simulink model "NewModel_v2"  (R2020a)
settings: Solver=VariableStepAuto  StartTime=0.0  StopTime=1000  FixedStep=0.1  RelTol=1e-3
values from neighbouring files (symbols this model uses):
  Ctr = 1.6    [ACC_DATA.m]
  F_aero = 1/(2*m_Follower)*Ro_A_Cd    (= 0.00026)    [ACC_DATA.m]
  F_grav = g*sin(theta)    [ACC_DATA.m]
  F_res = g*Cr*cos(theta)    [ACC_DATA.m]
  Kb = 0.08    [ACC_DATA.m]
  Kc = 1    [ACC_DATA.m]
  m_Follower = 1500    [ACC_DATA.m]
  max_ac = 3    [ACC_DATA.m]
  min_ac = -3    [ACC_DATA.m]
  r = 0.326    [ACC_DATA.m]
  Rf = 3.28    [ACC_DATA.m]
  Rtr = 1    [ACC_DATA.m]
  Tmax = 528.7 + 0.152*Ne - 0.0000217*Ne^2    (= 789.5)    [ACC_DATA.m]
  Ts = 0.1    [ACC_DATA.m]
  v0_lead = 20    [ACC_DATA.m]
  verr_gain = 0.4    [ACC_DATA.m]
  vx_gain = 0.1    [ACC_DATA.m]
  x0_ego = 10    [ACC_DATA.m]
  x0_lead = 500    [ACC_DATA.m]
  xerr_gain = 0.8    [ACC_DATA.m]
undefined symbols (not defined in the file or in its folder): sigbuilder_block
libraries: simulink x5
settings Model: SimulationMode=accelerator  Creator=91968  LastModifiedBy=91968

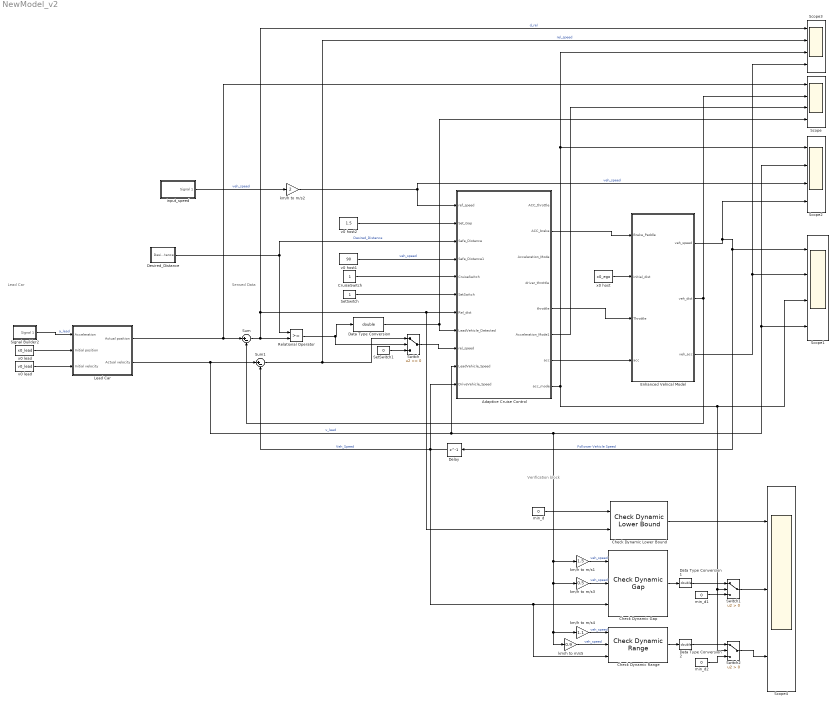
== system NewModel_v2 ==
  note: Verification block
  note: Lead Car
  note: Sensed Data
  Adaptive Cruise Control : Subsystem
  Check Dynamic Gap : simulink/Model Verification/Check  Dynamic Gap  Description=u < min || max < u  enabled=on  stopWhenAssertionFail=off  export=on  icon=graphic
      settings: SourceProductBaseCode=SL
  Check Dynamic Range : simulink/Model Verification/Check  Dynamic Range  Description=min < u < max  enabled=on  stopWhenAssertionFail=off  export=on  icon=graphic
      settings: SourceProductBaseCode=SL
  Check Dynamic Lower Bound : simulink/Model Verification/Check Dynamic  Lower Bound  Description=min < u  Enabled=on  stopWhenAssertionFail=off  export=on  icon=graphic
      settings: SourceProductBaseCode=SL
  CruiseSwitch : Constant
  Data Type Conversion : DataTypeConversion  OutDataTypeStr=double
  Data Type Conversion1 : DataTypeConversion  OutDataTypeStr=double
  Data Type Conversion2 : DataTypeConversion  OutDataTypeStr=double
  Delay : Delay  DelayLength=1  InitialCondition=0
  Desired_Distance : Subsystem  mask{Desired_Distance=10.0}
      mask DialogControl DescGroupVar Prompt: Set Desired Distance
      mask Display: image('C:\Users\Talha Rao\Pictures\070558928_iconm (2).jpeg');
  Enhanced Vehical Model : Subsystem
  Lead Car : Subsystem
  Relational Operator : RelationalOperator  OutDataTypeStr=boolean  RndMeth=Simplest
  Scope{,1..3} (4 alike) : Scope  NumInputPorts=4
  Scope4 : Scope  NumInputPorts=3
  SetSwitch : Constant
  SetSwitch1 : Constant  Value=0
  Signal Builder2 : Subsystem  Tag=STV Subsys  LoadFcn=sigbuilder_block('load');  StartFcn=sigbuilder_block('start');  StopFcn=sigbuilder_block('stop');  ClipboardFcn=sigbuilder_block('clipboard');  mask(Sigbuilder block){tuvar=[0:10]}
      mask help: Simulink:masks:SigbuilderBlock_MD
      mask init:
      | if ~strcmp(get_param(bdroot(gcbh),'SimulationStatus'),'stopped') tuvar = sigbuilder_block('maskInit'); end
      settings: CopyFcn=sigbuilder_block('copy');  DeleteFcn=sigbuilder_block('delete');  ModelCloseFcn=sigbuilder_block('modelClose');  PreSaveFcn=sigbuilder_block('preSave');  PauseFcn=sigbuilder_block('pause');  ContinueFcn=sigbuilder_block('continue');  NameChangeFcn=sigbuilder_block('namechange');  OpenFcn=sigbuilder_block('open',[-1359 225 891.75 468.75 ]);  CloseFcn=sigbuilder_block('close');
      mask Display: plot(0, 0, 100, 100,[2, 2, 32, 32, 2], [68, 8, 8, 68, 68],[32, 2], [38, 38], [32, 19, 2],[53, 60, 44], [32, 17, 17, 2],[16, 16, 31, 31]);txt = getActiveGroup(gcbh);text(2, 100, txt,'verticalAlignment', 'top');
  Sum : Sum  Inputs=|+-
  Sum1 : Sum  Inputs=|+-
  Switch : Switch  SaturateOnIntegerOverflow=on  InputSameDT=on
  Switch1 : Switch  Criteria=u2 > Threshold  SaturateOnIntegerOverflow=on  InputSameDT=on
  Switch2 : Switch  Criteria=u2 > Threshold  SaturateOnIntegerOverflow=on  InputSameDT=on
  input_speed : Subsystem  Tag=STV Subsys  LoadFcn=sigbuilder_block('load');  StartFcn=sigbuilder_block('start');  StopFcn=sigbuilder_block('stop');  ClipboardFcn=sigbuilder_block('clipboard');  mask(Sigbuilder block){tuvar=[0:10]}
      mask help: Simulink:masks:SigbuilderBlock_MD
      mask init:
      | if ~strcmp(get_param(bdroot(gcbh),'SimulationStatus'),'stopped') tuvar = sigbuilder_block('maskInit'); end
      settings: CopyFcn=sigbuilder_block('copy');  DeleteFcn=sigbuilder_block('delete');  ModelCloseFcn=sigbuilder_block('modelClose');  PreSaveFcn=sigbuilder_block('preSave');  PauseFcn=sigbuilder_block('pause');  ContinueFcn=sigbuilder_block('continue');  NameChangeFcn=sigbuilder_block('namechange');  OpenFcn=sigbuilder_block('open',[0 36 1440 716.25 ]);  CloseFcn=sigbuilder_block('close');
      mask Display: plot(0, 0, 100, 100,[2, 2, 32, 32, 2], [68, 8, 8, 68, 68],[32, 2], [38, 38], [32, 19, 2],[53, 60, 44], [32, 17, 17, 2],[16, 16, 31, 31]);txt = getActiveGroup(gcbh);text(2, 100, txt,'verticalAlignment', 'top');
  km/h to m/s1 : Gain  Gain=1.5
  km/h to m/s2 : Gain  Gain=2
  km/h to m/s3 : Gain  Gain=0.5
  km/h to m/s4 : Gain  Gain=1.1
  km/h to m/s5 : Gain  Gain=0.9
  min_d : Constant  Value=0
  min_d1 : Constant  Value=0
  min_d2 : Constant  Value=0
  v0 host1 : Constant  Value=90  SampleTime=Ts
  v0 host2 : Constant  Value=1.5  SampleTime=Ts
  v0 lead : Constant  Value=v0_lead  SampleTime=Ts
  x0 host : Constant  Value=x0_ego  SampleTime=Ts
  x0 lead : Constant  Value=x0_lead  SampleTime=Ts
  wires:
  x0 lead/1 -> Lead Car/2(Initial position)
  v0 lead/1 -> Lead Car/3(Initial velocity)
  Signal Builder2/1(Signal 1) -> Lead Car/1(Acceleration)  "a_lead"
  Lead Car/1(Actual position) -> Scope/1, Sum/1
  Lead Car/2(Actual velocity) -> Scope2/2, Scope1/4, km/h to m/s4/1, km/h to m/s5/1, km/h to m/s3/1, km/h to m/s1/1, Adaptive Cruise Control/10(LeadVehicle_Speed), Sum1/1  "v_lead"
  Delay/1 -> Check Dynamic Range/3, Check Dynamic Gap/3, Sum1/2, Adaptive Cruise Control/11(DriveVehicle_Speed)  "Veh_Speed"
  Desired_Distance/1(Desired_Distance) -> Relational Operator/1, Adaptive Cruise Control/3(Safe_Distance)  "Desired_Distance"
  Enhanced Vehical Model/1(veh_speed) -> Scope2/4, Delay/1, Scope1/1  "Follower Vehicle Speed"
  Sum/1 -> Scope3/1, Check Dynamic Lower Bound/2, Adaptive Cruise Control/7(Rel_dist), Relational Operator/2  "d_rel"
  x0 host/1 -> Enhanced Vehical Model/2(initial_dist)
  Enhanced Vehical Model/2(veh_dist) -> Scope/2, Sum/2
  v0 host2/1 -> Adaptive Cruise Control/2(Set_Gap)
  CruiseSwitch/1 -> Adaptive Cruise Control/5(CruiseSwitch)
  SetSwitch/1 -> Adaptive Cruise Control/6(SetSwitch)
  Adaptive Cruise Control/2(ACC_brake) -> Enhanced Vehical Model/1(Brake_Peddle)
  Enhanced Vehical Model/3(veh_acc) -> Scope3/4, Scope1/2
  input_speed/1(Signal 1) -> km/h to m/s2/1  "veh_speed"
  Adaptive Cruise Control/5(throttle) -> Enhanced Vehical Model/3(Throttle)
  Adaptive Cruise Control/6(Acceleration_Mode1) -> Scope/3
  Sum1/1 -> Switch/1, Scope3/2  "rel_speed"
  Relational Operator/1 -> Switch/2, Data Type Conversion/1
  Data Type Conversion/1 -> Scope/4, Adaptive Cruise Control/8(LeadVehicle_Detected)
  km/h to m/s2/1 -> Scope2/3, Adaptive Cruise Control/1(ref_speed)  "veh_speed"
  Switch/1 -> Adaptive Cruise Control/9(rel_speed)
  SetSwitch1/1 -> Switch/3
  v0 host1/1 -> Adaptive Cruise Control/4(Safe_Distance1)  "veh_speed"
  Adaptive Cruise Control/7(acc) -> Enhanced Vehical Model/4(acc)
  Adaptive Cruise Control/8(acc_mode) -> Scope1/3, Switch2/2, Switch1/2, Scope3/3, Scope2/1
  Check Dynamic Lower Bound/1 -> Scope4/1
  min_d/1 -> Check Dynamic Lower Bound/1
  min_d1/1 -> Switch1/3
  Check Dynamic Gap/1 -> Data Type Conversion1/1
  km/h to m/s1/1 -> Check Dynamic Gap/1  "veh_speed"
  km/h to m/s3/1 -> Check Dynamic Gap/2  "veh_speed"
  Switch1/1 -> Scope4/2
  Data Type Conversion1/1 -> Switch1/1
  km/h to m/s4/1 -> Check Dynamic Range/1  "veh_speed"
  km/h to m/s5/1 -> Check Dynamic Range/2  "veh_speed"
  Check Dynamic Range/1 -> Data Type Conversion2/1
  min_d2/1 -> Switch2/3
  Data Type Conversion2/1 -> Switch2/1
  Switch2/1 -> Scope4/3

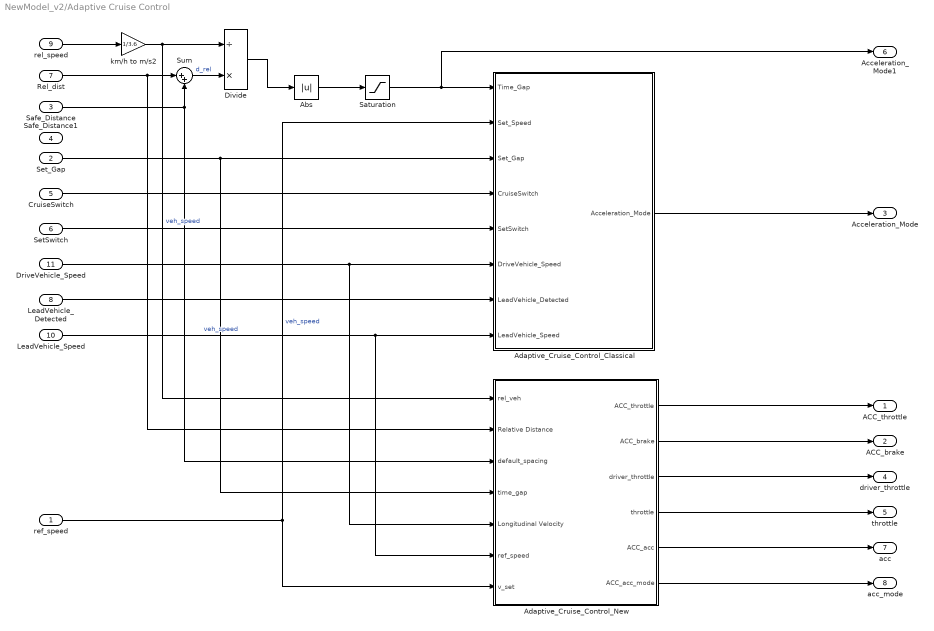
== system NewModel_v2/Adaptive Cruise Control ==
  ref_speed : Inport
  Set_Gap : Inport  Port=2
  Safe_Distance : Inport  Port=3
  Safe_Distance1 : Inport  Port=4
  CruiseSwitch : Inport  Port=5
  SetSwitch : Inport  Port=6
  Rel_dist : Inport  Port=7
  LeadVehicle_Detected : Inport  Port=8  OutMin=0  OutMax=1
  rel_speed : Inport  Port=9  OutMin=0  OutMax=1
  LeadVehicle_Speed : Inport  Port=10  OutMin=0  OutMax=255
  DriveVehicle_Speed : Inport  Port=11  OutMin=0  OutMax=255
  Abs : Abs
  Adaptive_Cruise_Control_Classical : Subsystem
  Adaptive_Cruise_Control_New : Subsystem
  Divide : Product  Inputs=/*
  Saturation : Saturate  UpperLimit=100  LowerLimit=0
  Sum : Sum  Inputs=|++
  km/h to m/s2 : Gain  Gain=1/3.6
  ACC_throttle : Outport
  ACC_brake : Outport  Port=2
  Acceleration_Mode : Outport  Port=3
  driver_throttle : Outport  Port=4
  throttle : Outport  Port=5
  Acceleration_Mode1 : Outport  Port=6
  acc : Outport  Port=7
  acc_mode : Outport  Port=8
  wires:
  SetSwitch/1 -> Adaptive_Cruise_Control_Classical/5(SetSwitch)
  Adaptive_Cruise_Control_Classical/1(Acceleration_Mode) -> Acceleration_Mode/1
  DriveVehicle_Speed/1 -> Adaptive_Cruise_Control_New/5(Longitudinal Velocity), Adaptive_Cruise_Control_Classical/6(DriveVehicle_Speed)
  Saturation/1 -> Acceleration_Mode1/1, Adaptive_Cruise_Control_Classical/1(Time_Gap)
  CruiseSwitch/1 -> Adaptive_Cruise_Control_Classical/4(CruiseSwitch)
  Set_Gap/1 -> Adaptive_Cruise_Control_New/4(time_gap), Adaptive_Cruise_Control_Classical/3(Set_Gap)
  LeadVehicle_Detected/1 -> Adaptive_Cruise_Control_Classical/7(LeadVehicle_Detected)
  Divide/1 -> Abs/1
  Rel_dist/1 -> Adaptive_Cruise_Control_New/2(Relative Distance), Sum/1
  rel_speed/1 -> km/h to m/s2/1
  Abs/1 -> Saturation/1
  Safe_Distance/1 -> Adaptive_Cruise_Control_New/3(default_spacing), Sum/2
  Sum/1 -> Divide/2  "d_rel"
  Adaptive_Cruise_Control_New/1(ACC_throttle) -> ACC_throttle/1
  Adaptive_Cruise_Control_New/2(ACC_brake) -> ACC_brake/1
  Adaptive_Cruise_Control_New/3(driver_throttle) -> driver_throttle/1
  Adaptive_Cruise_Control_New/4(throttle) -> throttle/1
  LeadVehicle_Speed/1 -> Adaptive_Cruise_Control_New/6(ref_speed), Adaptive_Cruise_Control_Classical/8(LeadVehicle_Speed)  "veh_speed"
  ref_speed/1 -> Adaptive_Cruise_Control_New/7(v_set), Adaptive_Cruise_Control_Classical/2(Set_Speed)  "veh_speed"
  km/h to m/s2/1 -> Adaptive_Cruise_Control_New/1(rel_veh), Divide/1  "veh_speed"
  Adaptive_Cruise_Control_New/5(ACC_acc) -> acc/1
  Adaptive_Cruise_Control_New/6(ACC_acc_mode) -> acc_mode/1

== system NewModel_v2/Desired_Distance ==
  Constant : Constant  Value=Desired_Distance
  Desired_Distance : Outport  VectorParamsAs1DForOutWhenUnconnected=off
  wires:
  Constant/1 -> Desired_Distance/1

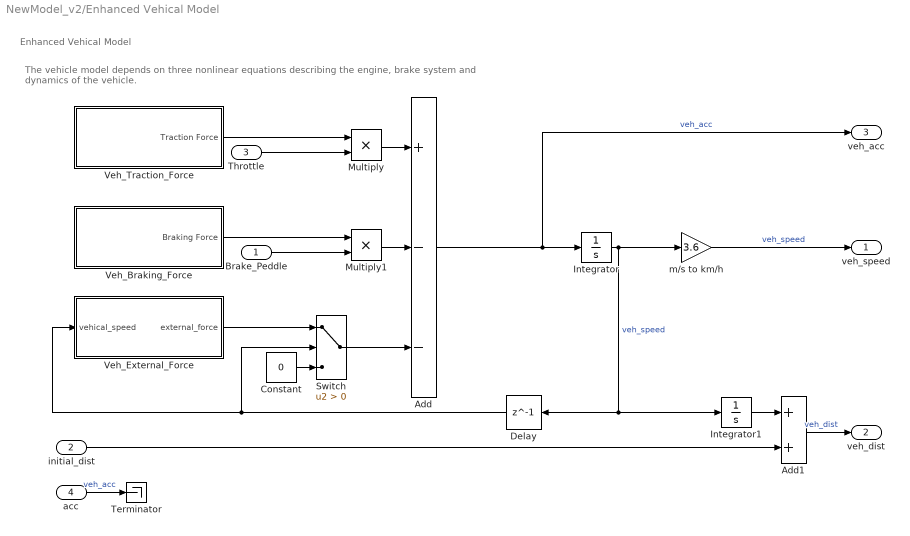
== system NewModel_v2/Enhanced Vehical Model ==
  note: The vehicle model depends on three nonlinear equations describing the engine, brake system and dynamics of the vehicle.
  note: Enhanced Vehical Model
  Brake_Peddle : Inport
  initial_dist : Inport  Port=2
  Throttle : Inport  Port=3
  acc : Inport  Port=4
  Add : Sum  Inputs=+--
  Add1 : Sum
  Constant : Constant  Value=0
  Delay : Delay  DelayLength=1  InitialCondition=0
  Integrator : Integrator
  Integrator1 : Integrator
  Multiply : Product
  Multiply1 : Product
  Switch : Switch  Criteria=u2 > Threshold  SaturateOnIntegerOverflow=on  InputSameDT=on
  Terminator : Terminator
  Veh_Braking_Force : Subsystem
  Veh_External_Force : Subsystem
  Veh_Traction_Force : Subsystem
  m/s to km/h : Gain  Gain=3.6
  veh_speed : Outport  VectorParamsAs1DForOutWhenUnconnected=off
  veh_dist : Outport  Port=2  VectorParamsAs1DForOutWhenUnconnected=off
  veh_acc : Outport  Port=3  VectorParamsAs1DForOutWhenUnconnected=off
  wires:
  Switch/1 -> Add/3
  Brake_Peddle/1 -> Multiply1/2
  Veh_Braking_Force/1("Braking Force ") -> Multiply1/1
  Multiply1/1 -> Add/2
  Multiply/1 -> Add/1
  Veh_Traction_Force/1(Traction Force) -> Multiply/1
  Integrator/1 -> m/s to km/h/1, Integrator1/1, Delay/1  "veh_speed"
  Integrator1/1 -> Add1/1
  Add1/1 -> veh_dist/1  "veh_dist"
  initial_dist/1 -> Add1/2
  Delay/1 -> Switch/2, Veh_External_Force/1(vehical_speed)
  Veh_External_Force/1(external_force) -> Switch/1
  Constant/1 -> Switch/3
  Throttle/1 -> Multiply/2
  m/s to km/h/1 -> veh_speed/1  "veh_speed"
  Add/1 -> veh_acc/1, Integrator/1  "veh_acc"
  acc/1 -> Terminator/1  "veh_acc"

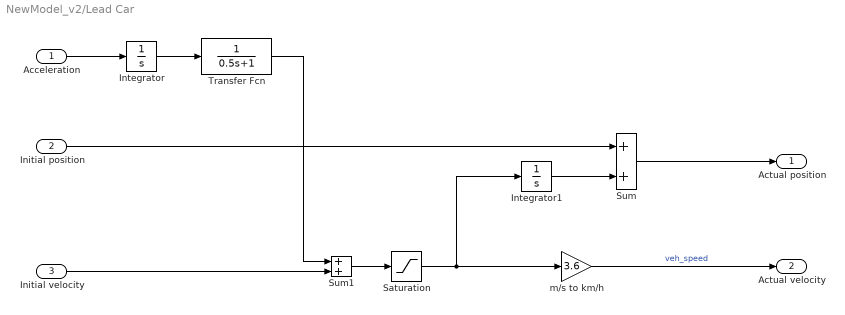
== system NewModel_v2/Lead Car ==
  Acceleration : Inport
  Initial position : Inport  Port=2
  Initial velocity : Inport  Port=3
  Integrator : Integrator
  Integrator1 : Integrator
  Saturation : Saturate  UpperLimit=200  LowerLimit=0
  Sum : Sum
  Sum1 : Sum
  Transfer Fcn : TransferFcn  Denominator=[0.5 1]
  m/s to km/h : Gain  Gain=3.6
  Actual position : Outport  VectorParamsAs1DForOutWhenUnconnected=off
  Actual velocity : Outport  Port=2  VectorParamsAs1DForOutWhenUnconnected=off
  wires:
  Transfer Fcn/1 -> Sum1/1
  Initial velocity/1 -> Sum1/2
  Integrator/1 -> Transfer Fcn/1
  Sum1/1 -> Saturation/1
  Acceleration/1 -> Integrator/1
  Initial position/1 -> Sum/1
  Integrator1/1 -> Sum/2
  Saturation/1 -> Integrator1/1, m/s to km/h/1
  Sum/1 -> Actual position/1
  m/s to km/h/1 -> Actual velocity/1  "veh_speed"

== system NewModel_v2/Signal Builder2 ==
  Demux : Demux  Tag=STV Demux  Outputs=1
      settings: DisplayOption=none
  FromWs : FromWorkspace  Tag=STV FromWs  VariableName=tuvar
      SigBuilderData=|
      | common.afterFinalStr = 'Extrapolate'
      | common.sampleTime = 0
      | dataSet.timeRange = [0 1000]
      | dataSet.name = 'Group 1'
      | sbobj.Groups.Name = 'Group 1'
      | sbobj.Groups.Signals.Name = 'Signal 1'
      | sbobj.Groups.Signals.XData = [0 20 30 40 60 80 100 126 150 200 250 300 350 400 451 502 539 549 599 650 700 749 799 847 902 956 1000]
      | sbobj.Groups.Signals.YData = [0.07 0.14 0.25 0.21 0.385 0.248 -0.09 0.032 0.006 -0.104 -0.092 -0.202 -0.182 -0.072 0.044 0.092 0.146 0.116 0.258 0.292 0.178 0.004 -0.132 -0.224 -0.124 -0.07 0]
      | sbobj.Groups.TimeRange = [0 1000]
  Signal 1 : Outport  Tag=STV Outport
  wires:
  Demux/1 -> Signal 1/1
  FromWs/1 -> Demux/1

== system NewModel_v2/input_speed ==
  Demux : Demux  Tag=STV Demux  Outputs=1
      settings: DisplayOption=none
  FromWs : FromWorkspace  Tag=STV FromWs  VariableName=tuvar
      SigBuilderData=|
      | common.afterFinalStr = 'Extrapolate'
      | common.sampleTime = 0
      | dataSet.timeRange = [0 1000]
      | dataSet.name = 'Group 1'
      | sbobj.Groups.Name = 'Group 1'
      | sbobj.Groups.Signals.Name = 'Signal 1'
      | sbobj.Groups.Signals.XData = [0 20 30 40 60 80 100 150 200 250 300 350 400 451 500 500 551 597 657 702 799 861 940 1000]
      | sbobj.Groups.Signals.YData = [0.5 6.6 10.6 15 22.8 31.2 33.6 52 69.4 76.4 69.2 62.4 60 45 28.4 27.8 37.2 55.2 62.2 61 52.2 54.8 75.4 56.2]
      | sbobj.Groups.TimeRange = [0 1000]
  Signal 1 : Outport  Tag=STV Outport
  wires:
  Demux/1 -> Signal 1/1
  FromWs/1 -> Demux/1

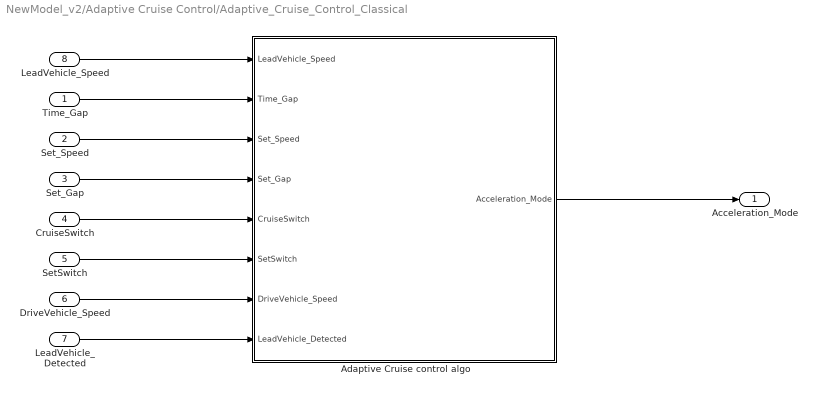
== system NewModel_v2/Adaptive Cruise Control/Adaptive_Cruise_Control_Classical ==
  Time_Gap : Inport
  Set_Speed : Inport  Port=2
  Set_Gap : Inport  Port=3
  CruiseSwitch : Inport  Port=4
  SetSwitch : Inport  Port=5
  DriveVehicle_Speed : Inport  Port=6  OutMin=0  OutMax=255
  LeadVehicle_Detected : Inport  Port=7  OutMin=0  OutMax=1
  LeadVehicle_Speed : Inport  Port=8  OutMin=0  OutMax=255
  Adaptive Cruise control algo : Stateflow chart  RequirementInfo={} %GIDa_57645b32_15f0_49df_b2ac_141007f7ec66  TreatAsAtomicUnit=on
  Acceleration_Mode : Outport  OutMin=0  OutMax=255
  wires:
  LeadVehicle_Speed/1 -> Adaptive Cruise control algo/1(LeadVehicle_Speed)
  Set_Gap/1 -> Adaptive Cruise control algo/4(Set_Gap)
  Set_Speed/1 -> Adaptive Cruise control algo/3(Set_Speed)
  Time_Gap/1 -> Adaptive Cruise control algo/2(Time_Gap)
  LeadVehicle_Detected/1 -> Adaptive Cruise control algo/8(LeadVehicle_Detected)
  DriveVehicle_Speed/1 -> Adaptive Cruise control algo/7(DriveVehicle_Speed)
  SetSwitch/1 -> Adaptive Cruise control algo/6(SetSwitch)
  CruiseSwitch/1 -> Adaptive Cruise control algo/5(CruiseSwitch)
  Adaptive Cruise control algo/1(Acceleration_Mode) -> Acceleration_Mode/1

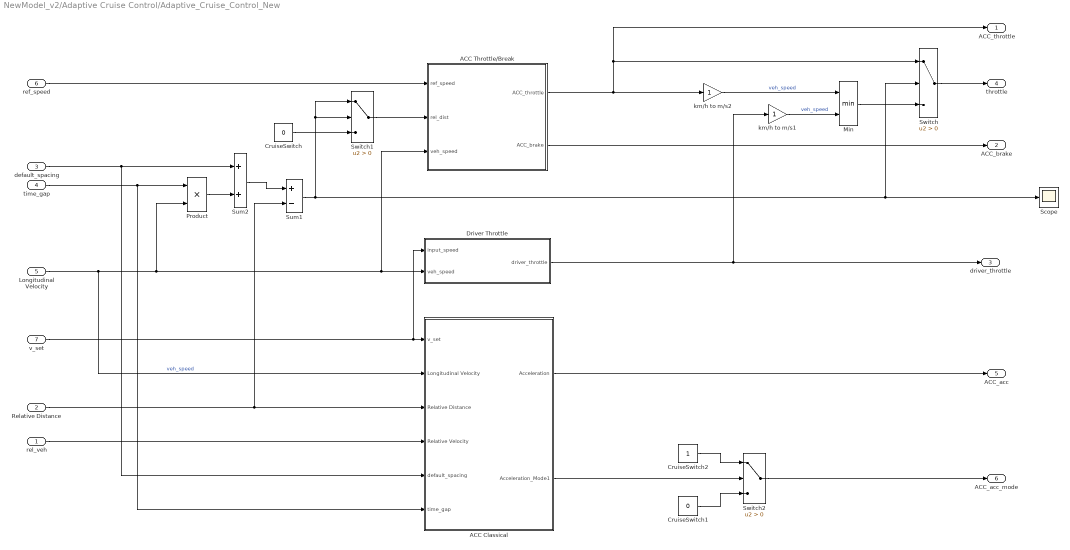
== system NewModel_v2/Adaptive Cruise Control/Adaptive_Cruise_Control_New ==
  rel_veh : Inport
  Relative Distance : Inport  Port=2
  default_spacing : Inport  Port=3
  time_gap : Inport  Port=4
  Longitudinal Velocity : Inport  Port=5
  ref_speed : Inport  Port=6
  v_set : Inport  Port=7
  ACC Classical : Subsystem  TreatAsAtomicUnit=on  VariantControl=controller_type == 1
      settings: RTWFileNameOpts=Use function name
  ACC Throttle/Break : Subsystem
  CruiseSwitch : Constant  Value=0
  CruiseSwitch1 : Constant  Value=0
  CruiseSwitch2 : Constant
  Driver Throttle : Subsystem
  Min : MinMax  Inputs=2
  Product : Product
  Scope : Scope
  Sum1 : Sum  Inputs=+-
  Sum2 : Sum
  Switch : Switch  Criteria=u2 > Threshold
  Switch1 : Switch  Criteria=u2 > Threshold
  Switch2 : Switch  Criteria=u2 > Threshold
  km/h to m/s1 : Gain
  km/h to m/s2 : Gain
  ACC_throttle : Outport
  ACC_brake : Outport  Port=2
  driver_throttle : Outport  Port=3
  throttle : Outport  Port=4
  ACC_acc : Outport  Port=5
  ACC_acc_mode : Outport  Port=6
  wires:
  ref_speed/1 -> ACC Throttle/Break/1(ref_speed)
  v_set/1 -> Driver Throttle/1(input_speed), ACC Classical/1(v_set)
  ACC Throttle/Break/2(ACC_brake) -> ACC_brake/1
  Relative Distance/1 -> Sum1/2, ACC Classical/3(Relative Distance)
  Driver Throttle/1(driver_throttle) -> km/h to m/s1/1, driver_throttle/1
  ACC Throttle/Break/1(ACC_throttle) -> km/h to m/s2/1, ACC_throttle/1, Switch/1
  Sum1/1 -> Switch1/1, Switch1/2, Scope/1, Switch/2
  Switch/1 -> throttle/1
  Sum2/1 -> Sum1/1
  default_spacing/1 -> ACC Classical/5(default_spacing), Sum2/1
  time_gap/1 -> ACC Classical/6(time_gap), Product/1
  Product/1 -> Sum2/2
  Longitudinal Velocity/1 -> Product/2, Driver Throttle/2(veh_speed), ACC Throttle/Break/3(veh_speed), ACC Classical/2(Longitudinal Velocity)  "veh_speed"
  Switch1/1 -> ACC Throttle/Break/2(rel_dist)
  CruiseSwitch/1 -> Switch1/3
  km/h to m/s2/1 -> Min/1  "veh_speed"
  km/h to m/s1/1 -> Min/2  "veh_speed"
  Min/1 -> Switch/3
  rel_veh/1 -> ACC Classical/4(Relative Velocity)
  ACC Classical/1(Acceleration) -> ACC_acc/1
  ACC Classical/2(Acceleration_Mode1) -> Switch2/2
  CruiseSwitch1/1 -> Switch2/3
  CruiseSwitch2/1 -> Switch2/1
  Switch2/1 -> ACC_acc_mode/1

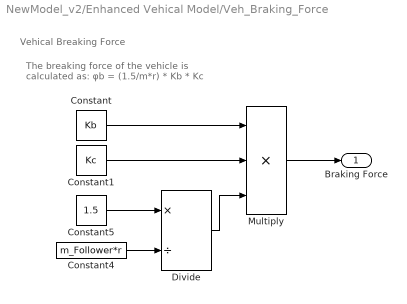
== system NewModel_v2/Enhanced Vehical Model/Veh_Braking_Force ==
  note: Vehical Breaking Force
  note: The breaking force of the vehicle is calculated as:
      | φb = (1.5/m*r) * Kb * Kc
  Constant : Constant  Value=Kb
  Constant1 : Constant  Value=Kc
  Constant4 : Constant  Value=m_Follower*r
  Constant5 : Constant  Value=1.5
  Divide : Product  Inputs=*/
  Multiply : Product  Inputs=3
  "Braking Force " : Outport  VectorParamsAs1DForOutWhenUnconnected=off
  wires:
  Multiply/1 -> "Braking Force "/1
  Constant4/1 -> Divide/2
  Constant1/1 -> Multiply/2
  Constant/1 -> Multiply/1
  Constant5/1 -> Divide/1
  Divide/1 -> Multiply/3

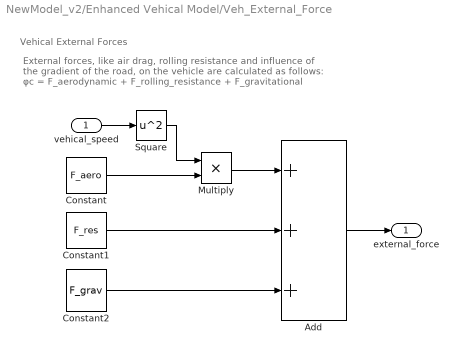
== system NewModel_v2/Enhanced Vehical Model/Veh_External_Force ==
  note: External forces, like air drag, rolling resistance and
      | influence of the gradient of the road, on the vehicle are calculated as follows:
      |
      | φc = F_aerodynamic + F_rolling_resistance + F_gravitational
  note: Vehical External Forces
  vehical_speed : Inport
  Add : Sum  Inputs=+++
  Constant : Constant  Value=F_aero
  Constant1 : Constant  Value=F_res
  Constant2 : Constant  Value=F_grav
  Multiply : Product
  Square : Math  Operator=square  SignedPower=on  SaturateOnIntegerOverflow=on
  external_force : Outport  VectorParamsAs1DForOutWhenUnconnected=off
  wires:
  Add/1 -> external_force/1
  Constant1/1 -> Add/2
  Constant2/1 -> Add/3
  Constant/1 -> Multiply/2
  vehical_speed/1 -> Square/1
  Square/1 -> Multiply/1
  Multiply/1 -> Add/1

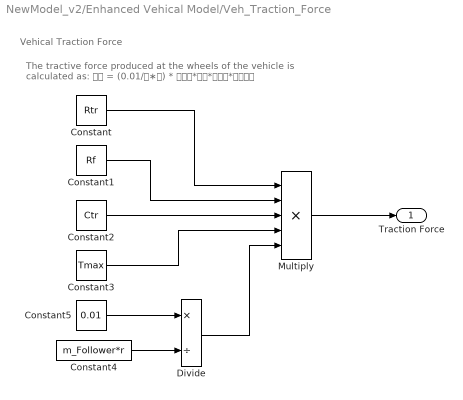
== system NewModel_v2/Enhanced Vehical Model/Veh_Traction_Force ==
  note: The tractive force produced at the wheels of the vehicle is calculated as:
      | 𝜑𝑡 = (0.01/𝑚∗𝑟) * 𝑅𝑡𝑟*𝑅𝑓*𝐶𝑡𝑟*𝑇𝑚𝑎𝑥
  note: Vehical Traction Force
  Constant : Constant  Value=Rtr
  Constant1 : Constant  Value=Rf
  Constant2 : Constant  Value=Ctr
  Constant3 : Constant  Value=Tmax
  Constant4 : Constant  Value=m_Follower*r
  Constant5 : Constant  Value=0.01
  Divide : Product  Inputs=*/
  Multiply : Product  Inputs=5
  Traction Force : Outport  VectorParamsAs1DForOutWhenUnconnected=off
  wires:
  Constant/1 -> Multiply/1
  Constant4/1 -> Divide/2
  Constant1/1 -> Multiply/2
  Constant5/1 -> Divide/1
  Constant3/1 -> Multiply/4
  Divide/1 -> Multiply/5
  Constant2/1 -> Multiply/3
  Multiply/1 -> Traction Force/1

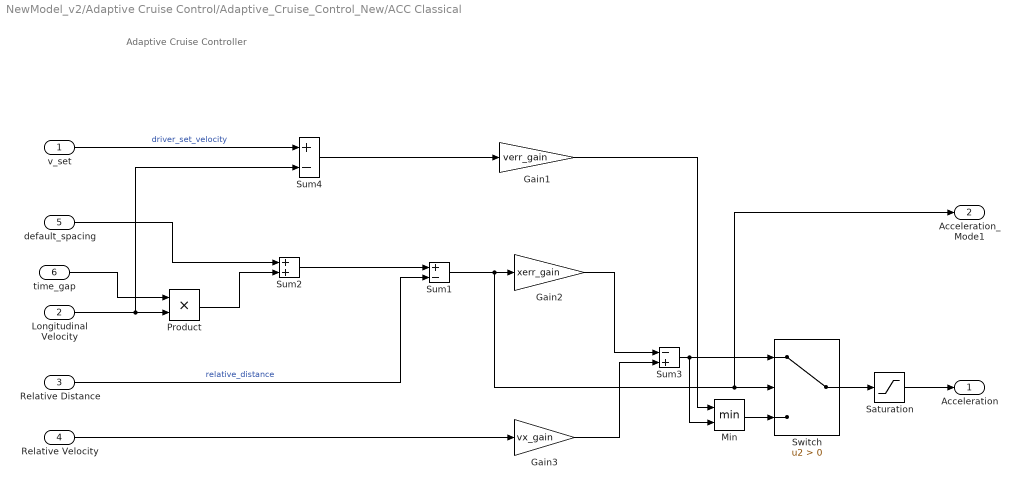
== system NewModel_v2/Adaptive Cruise Control/Adaptive_Cruise_Control_New/ACC Classical ==
  note: Adaptive Cruise Controller
  v_set : Inport
  Longitudinal Velocity : Inport  Port=2
  Relative Distance : Inport  Port=3
  Relative Velocity : Inport  Port=4
  default_spacing : Inport  Port=5
  time_gap : Inport  Port=6
  Gain1 : Gain  Gain=verr_gain
  Gain2 : Gain  Gain=xerr_gain
  Gain3 : Gain  Gain=vx_gain
  Min : MinMax  Inputs=2
  Product : Product
  Saturation : Saturate  UpperLimit=max_ac  LowerLimit=min_ac
  Sum1 : Sum  Inputs=+-
  Sum2 : Sum
  Sum3 : Sum  Inputs=-+
  Sum4 : Sum  Inputs=+-
  Switch : Switch  Criteria=u2 > Threshold
  Acceleration : Outport  VectorParamsAs1DForOutWhenUnconnected=off
  Acceleration_Mode1 : Outport  Port=2  VectorParamsAs1DForOutWhenUnconnected=off
  wires:
  Longitudinal Velocity/1 -> Product/2, Sum4/2
  default_spacing/1 -> Sum2/1
  Gain2/1 -> Sum3/1
  Sum4/1 -> Gain1/1
  Min/1 -> Switch/3
  Gain3/1 -> Sum3/2
  Switch/1 -> Saturation/1
  Relative Velocity/1 -> Gain3/1
  time_gap/1 -> Product/1
  Saturation/1 -> Acceleration/1
  Product/1 -> Sum2/2
  v_set/1 -> Sum4/1  "driver_set_velocity"
  Sum3/1 -> Min/2, Switch/1
  Sum1/1 -> Acceleration_Mode1/1, Switch/2, Gain2/1
  Gain1/1 -> Min/1
  Relative Distance/1 -> Sum1/2  "relative_distance"
  Sum2/1 -> Sum1/1

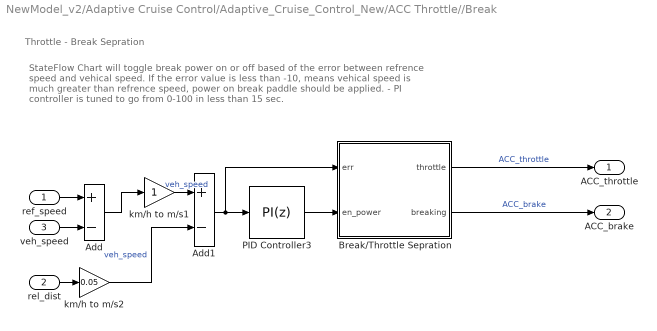
== system NewModel_v2/Adaptive Cruise Control/Adaptive_Cruise_Control_New/ACC Throttle//Break ==
  note: StateFlow Chart will toggle break power on or off based of the error between refrence speed and
      | vehical speed. If the error value is less than -10, means vehical speed is much greater than refrence
      | speed, power on break paddle should be applied.
      |
      | - PI controller is tuned to go from 0-100 in less than 15 sec.
  note: Throttle - Break Sepration
  ref_speed : Inport
  rel_dist : Inport  Port=2
  veh_speed : Inport  Port=3
  Add : Sum  Inputs=+-
  Add1 : Sum  Inputs=+-
  Break/Throttle Sepration : Stateflow chart  TreatAsAtomicUnit=on
  PID Controller3 : simulink/Continuous/PID Controller  Controller=PI  Form=Parallel  TimeDomain=Discrete-time  UseExternalTs=off  SampleTime=0.02  IntegratorMethod=Trapezoidal  FilterMethod=Forward Euler  ControllerParametersSource=internal  P=5  I=2  D=1  UseFilter=on  N=100  TunerSelectOption=Transfer Function Based (PID Tuner App)  InitialConditionSource=internal  InitialConditionForIntegrator=0  InitialConditionForFilter=0  DifferentiatorICPrevScaledInput=0  ExternalReset=none  TrackingMode=off  Kt=1  LimitOutput=on  UpperSaturationLimit=100  LowerSaturationLimit=-100  LinearizeAsGain=on  AntiWindupMode=clamping  Kb=1  POutMin=[]  POutMax=[]  IOutMin=[]  IOutMax=[]  DOutMin=[]  DOutMax=[]  NOutMin=[]  NOutMax=[]  SumOutMin=[]  SumOutMax=[]  SaturationOutMin=[]  SaturationOutMax=[]  PParamMin=[]  PParamMax=[]  IParamMin=[]  IParamMax=[]  DParamMin=[]  DParamMax=[]  NParamMin=[]  NParamMax=[]  KbParamMin=[]  KbParamMax=[]  KtParamMin=[]  KtParamMax=[]  KbOutMin=[]  KbOutMax=[]  KtOutMin=[]  KtOutMax=[]  IntegratorOutMin=[]  IntegratorOutMax=[]  FilterOutMin=[]  FilterOutMax=[]  SumI1OutMin=[]  SumI1OutMax=[]  SumI2OutMin=[]  SumI2OutMax=[]  SumI3OutMin=[]  SumI3OutMax=[]  SumI4OutMin=[]  SumI4OutMax=[]  SumDOutMin=[]  SumDOutMax=[]  DifferentiatorOutMin=[]  DifferentiatorOutMax=[]  FilterDiffOutCoefMin=[]  FilterDiffOutCoefMax=[]  ReciprocalOutMin=[]  ReciprocalOutMax=[]  SumDenOutMin=[]  SumDenOutMax=[]  SumNumOutMin=[]  SumNumOutMax=[]  DivideOutMin=[]  DivideOutMax=[]  UdiffTsProdOutMin=[]  UdiffTsProdOutMax=[]  NTsProdOutMin=[]  NTsProdOutMax=[]  UintegralTsProdOutMin=[]  UintegralTsProdOutMax=[]  UngainTsProdOutMin=[]  UngainTsProdOutMax=[]  IntegratorContinuousStateAttributes=''  IntegratorStateMustResolveToSignalObject=off  IntegratorRTWStateStorageClass=Auto  FilterContinuousStateAttributes=''  FilterStateMustResolveToSignalObject=off  FilterRTWStateStorageClass=Auto  ParallelPVariant=InternalParameters  IdealPVariant=Disabled  IVariant=InternalParameters  DVariant=Disabled  IntegratorVariant=Discrete  SatVariant=Enabled  AWVariant=DiscClampingParallel  PCopyVariant=Disabled  TRVariant=Disabled  FdbkBlocksVariant=Feedback  IdealPFdbkVariant=Passthrough  SatFdbkVariant=Passthrough  DerivativeFilterVariant=Disabled  NVariant=Disabled  NCopyVariant=Disabled_SignalSpec  FilterICVariant=Disabled  IntegratorICVariant=InternalICs  ExternalResetVariant=Disabled  TRSumVariant=Passthrough  SumFdbkVariant=Enabled  SumVariant=Sum_PI  TsampFilterVariant=InternalTs  TsampNgainVariant=Passthrough  TsampIntegralVariant=Passthrough
  km/h to m/s1 : Gain
  km/h to m/s2 : Gain  Gain=0.05
  ACC_throttle : Outport  VectorParamsAs1DForOutWhenUnconnected=off
  ACC_brake : Outport  Port=2  VectorParamsAs1DForOutWhenUnconnected=off
  wires:
  ref_speed/1 -> Add/1
  veh_speed/1 -> Add/2
  PID Controller3/1 -> Break/Throttle Sepration/2(en_power)
  Add1/1 -> Break/Throttle Sepration/1(err), PID Controller3/1
  Break/Throttle Sepration/1(throttle) -> ACC_throttle/1  "ACC_throttle"
  Break/Throttle Sepration/2(breaking) -> ACC_brake/1  "ACC_brake"
  Add/1 -> km/h to m/s1/1
  rel_dist/1 -> km/h to m/s2/1
  km/h to m/s2/1 -> Add1/2  "veh_speed"
  km/h to m/s1/1 -> Add1/1  "veh_speed"

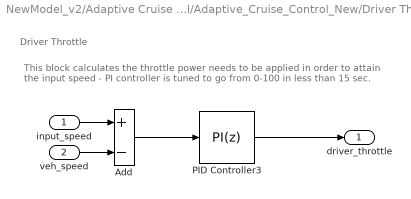
== system NewModel_v2/Adaptive Cruise Control/Adaptive_Cruise_Control_New/Driver Throttle ==
  note: This block calculates the throttle power needs to be applied in order to attain the input speed
      | - PI controller is tuned to go from 0-100 in less than 15 sec.
  note: Driver Throttle
  input_speed : Inport
  veh_speed : Inport  Port=2
  Add : Sum  Inputs=+-
  PID Controller3 : simulink/Continuous/PID Controller  Controller=PI  Form=Parallel  TimeDomain=Discrete-time  UseExternalTs=off  SampleTime=0.02  IntegratorMethod=Trapezoidal  FilterMethod=Forward Euler  ControllerParametersSource=internal  P=2  I=0.5  D=0  UseFilter=on  N=100  TunerSelectOption=Transfer Function Based (PID Tuner App)  InitialConditionSource=internal  InitialConditionForIntegrator=0  InitialConditionForFilter=0  DifferentiatorICPrevScaledInput=0  ExternalReset=none  TrackingMode=off  Kt=1  LimitOutput=on  UpperSaturationLimit=100  LowerSaturationLimit=-100  LinearizeAsGain=on  AntiWindupMode=clamping  Kb=1  POutMin=[]  POutMax=[]  IOutMin=[]  IOutMax=[]  DOutMin=[]  DOutMax=[]  NOutMin=[]  NOutMax=[]  SumOutMin=[]  SumOutMax=[]  SaturationOutMin=[]  SaturationOutMax=[]  PParamMin=[]  PParamMax=[]  IParamMin=[]  IParamMax=[]  DParamMin=[]  DParamMax=[]  NParamMin=[]  NParamMax=[]  KbParamMin=[]  KbParamMax=[]  KtParamMin=[]  KtParamMax=[]  KbOutMin=[]  KbOutMax=[]  KtOutMin=[]  KtOutMax=[]  IntegratorOutMin=[]  IntegratorOutMax=[]  FilterOutMin=[]  FilterOutMax=[]  SumI1OutMin=[]  SumI1OutMax=[]  SumI2OutMin=[]  SumI2OutMax=[]  SumI3OutMin=[]  SumI3OutMax=[]  SumI4OutMin=[]  SumI4OutMax=[]  SumDOutMin=[]  SumDOutMax=[]  DifferentiatorOutMin=[]  DifferentiatorOutMax=[]  FilterDiffOutCoefMin=[]  FilterDiffOutCoefMax=[]  ReciprocalOutMin=[]  ReciprocalOutMax=[]  SumDenOutMin=[]  SumDenOutMax=[]  SumNumOutMin=[]  SumNumOutMax=[]  DivideOutMin=[]  DivideOutMax=[]  UdiffTsProdOutMin=[]  UdiffTsProdOutMax=[]  NTsProdOutMin=[]  NTsProdOutMax=[]  UintegralTsProdOutMin=[]  UintegralTsProdOutMax=[]  UngainTsProdOutMin=[]  UngainTsProdOutMax=[]  IntegratorContinuousStateAttributes=''  IntegratorStateMustResolveToSignalObject=off  IntegratorRTWStateStorageClass=Auto  FilterContinuousStateAttributes=''  FilterStateMustResolveToSignalObject=off  FilterRTWStateStorageClass=Auto  ParallelPVariant=InternalParameters  IdealPVariant=Disabled  IVariant=InternalParameters  DVariant=Disabled  IntegratorVariant=Discrete  SatVariant=Enabled  AWVariant=DiscClampingParallel  PCopyVariant=Disabled  TRVariant=Disabled  FdbkBlocksVariant=Feedback  IdealPFdbkVariant=Passthrough  SatFdbkVariant=Passthrough  DerivativeFilterVariant=Disabled  NVariant=Disabled  NCopyVariant=Disabled_SignalSpec  FilterICVariant=Disabled  IntegratorICVariant=InternalICs  ExternalResetVariant=Disabled  TRSumVariant=Passthrough  SumFdbkVariant=Enabled  SumVariant=Sum_PI  TsampFilterVariant=InternalTs  TsampNgainVariant=Passthrough  TsampIntegralVariant=Passthrough
  driver_throttle : Outport  VectorParamsAs1DForOutWhenUnconnected=off
  wires:
  input_speed/1 -> Add/1
  veh_speed/1 -> Add/2
  PID Controller3/1 -> driver_throttle/1
  Add/1 -> PID Controller3/1

== stateflow chart NewModel_v2/Adaptive Cruise Control/Adaptive_Cruise_Control_New/ACC Throttle//Break/Break//Throttle Sepration ==
  note: Break/Throttle Separation
  note: State
      | Description
      | Condition
      | Next State
      |
      | OPEN_THROTTLE
      | Apply power on throttle when error is >= -10
      | err >= -10
      | APPLY_BREAK
      |
      | APPLY_BREAK
      | Apply power on break when error is < -10
      | err < -10
      | OPEN_THROTTLE
  state OPEN_THROTTLE
    en: breaking = 0;
    during: throttle = en_power;
  state APPLY_BREAK
    during: breaking = en_power;
    en:throttle = 0;
  (default) -> OPEN_THROTTLE
  OPEN_THROTTLE -> APPLY_BREAK : [err<-5]
  APPLY_BREAK -> OPEN_THROTTLE : [err >= 0]
  data: throttle output; breaking output; err input; en_power input

== stateflow chart NewModel_v2/Adaptive Cruise Control/Adaptive_Cruise_Control_Classical/Adaptive Cruise control algo ==
  state ACC_STANDBY_MODE
    entry:
    Acceleration_Mode = 1;
  state ACC_OFF_MODE
    entry:
    Acceleration_Mode = 0;
  state ACC_ON_MODE
    state LeadVehicle_Not_Detected_Resume
      entry:
      Acceleration_Mode= 1;
    state LeadVehicle_Detected_Resume
      entry:
      Acceleration_Mode= 3;
    state LeadVehicle_Detected_Follow
      entry:
      Acceleration_Mode= 2;
    state LeadVehicle_Not_Detected
      entry:
      Acceleration_Mode= 1;
    state LeadVehicle_Speed_equal_Set_Speed
      entry:
      Acceleration_Mode= 4;
    state LeadVehicle_Speed_lessthan_Set_Speed
      entry:
      Acceleration_Mode= 5;
    (default) -> LeadVehicle_Detected_Follow
    LeadVehicle_Detected_Resume -> LeadVehicle_Not_Detected_Resume [order 1] : [LeadVehicle_Detected ==0]
    LeadVehicle_Detected_Follow -> LeadVehicle_Detected_Resume [order 3] : [(DriveVehicle_Speed==Set_Speed) ...
        | && (LeadVehicle_Speed >= Set_Speed)...
        |  && (Time_Gap>=Set_Gap)]
    LeadVehicle_Speed_lessthan_Set_Speed -> LeadVehicle_Not_Detected_Resume [order 2] : [(LeadVehicle_Detected==0) ...
        | || (DriveVehicle_Speed <= Set_Speed)]
    LeadVehicle_Detected_Resume -> LeadVehicle_Speed_lessthan_Set_Speed [order 2] : [(DriveVehicle_Speed< Set_Speed) ...
        | && (LeadVehicle_Speed > DriveVehicle_Speed)...
        | || (Time_Gap >= Set_Gap)]
    LeadVehicle_Speed_lessthan_Set_Speed -> LeadVehicle_Detected_Resume [order 1] : [(DriveVehicle_Speed< Set_Speed) ...
        | && (LeadVehicle_Speed > DriveVehicle_Speed)...
        | && (Time_Gap >= Set_Gap)]
    LeadVehicle_Detected_Follow -> LeadVehicle_Not_Detected [order 2] : [LeadVehicle_Detected ==0]
    LeadVehicle_Not_Detected -> LeadVehicle_Detected_Follow [order 1] : [(LeadVehicle_Detected==1) && ...
        | (DriveVehicle_Speed == Set_Speed) && ...
        |  (LeadVehicle_Speed >= Set_Speed) &&...
        |  (Time_Gap>=Set_Gap)]
    LeadVehicle_Detected_Follow -> LeadVehicle_Speed_equal_Set_Speed [order 1] : [(LeadVehicle_Detected==1) && ((LeadVehicle_Speed < Set_Speed) || (Time_Gap<Set_Gap))]
    LeadVehicle_Speed_equal_Set_Speed -> LeadVehicle_Not_Detected [order 1] : [(LeadVehicle_Detected==0) && ...
        | (DriveVehicle_Speed == Set_Speed)]
    LeadVehicle_Not_Detected -> LeadVehicle_Speed_equal_Set_Speed [order 2] : [(LeadVehicle_Detected==1) && ...
        | (LeadVehicle_Speed < Set_Speed) || ...
        | (Time_Gap<Set_Gap)]
    LeadVehicle_Speed_lessthan_Set_Speed -> LeadVehicle_Speed_equal_Set_Speed [order 3] : [(LeadVehicle_Speed< Set_Speed) ...
        | && (LeadVehicle_Speed < DriveVehicle_Speed)...
        | || (Time_Gap == 0.75*Set_Gap)]
    LeadVehicle_Speed_equal_Set_Speed -> LeadVehicle_Speed_lessthan_Set_Speed [order 2] : [(LeadVehicle_Speed*1.25 >= DriveVehicle_Speed) ...
        | && (LeadVehicle_Speed*0.75 <= DriveVehicle_Speed)...
        | && (DriveVehicle_Speed < Set_Speed) && (Time_Gap <=1.25*Set_Gap)...
        | && (Time_Gap >= 0.75*Set_Gap)]
  note: State
      | Description
      | Condition
      | Next State
      |
      | IDLE_STATE
      | Set cc refrence speed & set_speed equal to input speed
      | default || ACC_OFF
      | SPEED_TRACKING
      |
      | SPEED_TRACKING
      | Follow the set speed chosen by the driver
      | ACC_ON event occured && obstacle_distance < set_distance
      | DISTANCE_TRACKING / IDLE_STATE
      |
      | DISTANCE_TRACKING
      | Follow the tracking speed to keep the min distance maintained
      | obstacle_distance > set_distance...
      | && after(60,sec)
      | SPEED_TRACKING
  (default) -> ACC_OFF_MODE
  ACC_OFF_MODE -> ACC_STANDBY_MODE : [CruiseSwitch == 1]
  ACC_STANDBY_MODE -> ACC_OFF_MODE [order 1] : [CruiseSwitch==0]
  ACC_ON_MODE -> ACC_STANDBY_MODE [order 1] : [SetSwitch ==0]
  ACC_STANDBY_MODE -> ACC_ON_MODE [order 2] : [SetSwitch ==1]
  ACC_ON_MODE -> ACC_OFF_MODE [order 2] : [CruiseSwitch == 0]
  data: LeadVehicle_Speed input; Time_Gap input; Set_Speed input; Set_Gap input; CruiseSwitch input [0..1]; SetSwitch input [0..1]; DriveVehicle_Speed input; LeadVehicle_Detected input; Acceleration_Mode output
